simulink model "muelle_simulink"  (R2014a)
settings: Solver=ode45  StartTime=0.0  StopTime=60.0  RelTol=1e-3
settings Model: Creator=emilio  LastModifiedBy=emilio

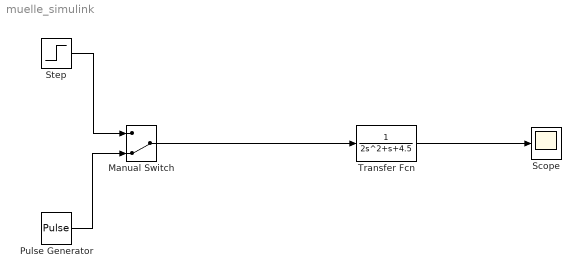
== system muelle_simulink ==
  Manual Switch : ManualSwitch  CurrentSetting=0
  Pulse Generator : DiscretePulseGenerator  PulseType=Time based  Period=30  PulseWidth=50  PhaseDelay=15
  Scope : Scope
      settings: TimeRange=10
  Step : Step  SampleTime=.5
  Transfer Fcn : TransferFcn  Denominator=[2, 1, 4.5]
  wires:
  Step/1 -> Manual Switch/1
  Manual Switch/1 -> Transfer Fcn/1
  Pulse Generator/1 -> Manual Switch/2
  Transfer Fcn/1 -> Scope/1
